simulink model "Control_Integral_simu"  (R2021a)
settings: Solver=VariableStepAuto  StartTime=0.0  StopTime=10.0  RelTol=1e-3
values from neighbouring files (symbols this model uses):
  A = [-2 -1; 0 -4]    [Control_Integral.m]    (also in Controlabilidad.m = P.a; Ejemplo_filminas.m = SS.A; Ejercicio_Inestable.m = [100, 0; 160, 200]; Ejercicio_Valvulas.m = double(A))
  B = [1; 0]    [Control_Integral.m]    (also in Controlabilidad.m = P.b; Ejemplo_filminas.m = SS.B; Ejercicio_Inestable.m = [70; 160]; Ejercicio_Valvulas.m = double(B))
  C = [1 1]    [Control_Integral.m]    (also in Controlabilidad.m = P.c; Ejemplo_filminas.m = SS.C; Ejercicio_Inestable.m = [1, 1]; Ejercicio_Valvulas.m = double(C))
  D = 0    [Control_Integral.m]    (also in Controlabilidad.m = P.d; Ejemplo_filminas.m = SS.D; Ejercicio_Inestable.m = 1; Ejercicio_Valvulas.m = double(D))
  ki = 10    [Control_Integral.m]    (also in Ejemplo_filminas.m = - Ka(end); Ejercicio_Inestable.m = - Ka(end); Ejercicio_Valvulas.m = - Ka(end))
settings Model: Creator=Santiago  LastModifiedBy=Santiago

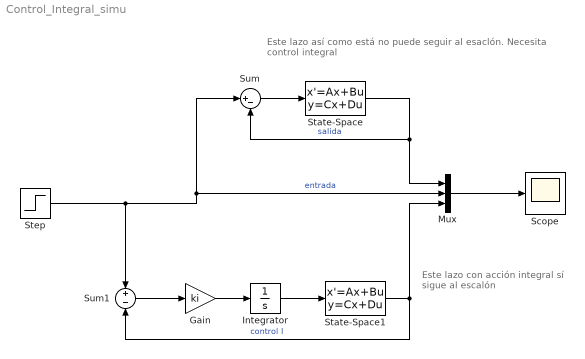
== system Control_Integral_simu ==
  note: Este lazo con acción integral
      | sí sigue al escalón
  note: Este lazo así como está no puede seguir al esaclón.
      | Necesita control integral
  Gain : Gain  Gain=ki
  Integrator : Integrator
  Mux : Mux  Inputs=3
  Scope : Scope
  State-Space : StateSpace  A=A  B=B  C=C  D=D  InitialCondition=0
  State-Space1 : StateSpace  A=A  B=B  C=C  D=D  InitialCondition=0
  Step : Step  SampleTime=0
  Sum : Sum  Inputs=|+-
  Sum1 : Sum  Inputs=+|-
  wires:
  Step/1 -> Sum1/1, Mux/2, Sum/1  "entrada"
  Sum/1 -> State-Space/1
  State-Space/1 -> Mux/1, Sum/2  "salida"
  Mux/1 -> Scope/1
  Integrator/1 -> State-Space1/1
  State-Space1/1 -> Mux/3, Sum1/2  "control I"
  Sum1/1 -> Gain/1
  Gain/1 -> Integrator/1
